simulink model "Model_TranslationEngine64"  (R2022b)
settings: Solver=FixedStepDiscrete  StartTime=0.0  StopTime=5  RelTol=1e-3  EnableMultiTasking=on
InitFcn:
  | % Initialize model
  | ModelSettings=BTConfig.GetModelSettings();
  | 
  | ModelSettings.Validate();
  | 
  | ModelInit;
  | 
  | 
  | % load library data
  | GainLibrary_data;
  | % Load saved values from partition process
  | CapturedConstMask.LoadMapFromFile(bdroot)
StartFcn:
  | % make sure all the simulated RTC requests are found
  | %RTC_SIM_OBJ.ValidateREQs();
undefined symbols (not defined in the file or in its folder): AA, BPLP, Column, NumHFRefBPF, NumHFRefLPF, NumMusicChannels, Row, VolumeMuteConfig
libraries: TuneVar x925, TOP x490, FeaturePath x111, CapturedConstLib x52
(part 33 of 34)

== matlab function Model_TranslationEngine64/ModelPreAmp/DecRate/AudioPilot35/Audiopilot_3_5/GainCalculation/Boosts/DownwardExpansionOn/BassEnable ==
  data: on input; slopeOut output; slope input
  events: trigger input FUNCTION_CALL_EVENT
function slopeOut  = enable(on,slope)
%#codegen
slopeOut = slope.Value * on.Value;

== matlab function Model_TranslationEngine64/ModelPreAmp/DecRate/AudioPilot35/Audiopilot_3_5/GainCalculation/Boosts/DownwardExpansionOn/MidrangeEnable ==
  data: on input; slopeOut output; slope input
  events: trigger input FUNCTION_CALL_EVENT
function slopeOut  = enable(on,slope)
%#codegen
slopeOut = slope.Value * on.Value;

== matlab function Model_TranslationEngine64/ModelPreAmp/DecRate/AudioPilot35/Audiopilot_3_5/GainApplication/Compensation/MidrangeLpfAlignDelay/AlignDelay/MaxCheck ==
  data: DelaySamples input; MaxDelaySamples input; Samples output
  events: trigger input FUNCTION_CALL_EVENT
function Samples = fcn(DelaySamples, MaxDelaySamples)
% Check that number of delay samples will not exceed allotted delay buffer

%Check against the max
if DelaySamples.Value > MaxDelaySamples
    TranslateError('Delay amount cannot be greater than specified max delay');
end

Samples = DelaySamples.Value;

== matlab function Model_TranslationEngine64/ModelPreAmp/DecRate/AudioPilot35/Audiopilot_3_5/GainCalculation/Boosts/DownwardExpansionOn/TrebleEnable ==
  data: on input; slopeOut output; slope input
  events: trigger input FUNCTION_CALL_EVENT
function slopeOut  = enable(on,slope)
%#codegen
slopeOut = slope.Value * on.Value;

== matlab function Model_TranslationEngine64/ModelPreAmp/DecRate/AudioPilot35/Audiopilot_3_5/GainCalculation/Boosts/DyneqOn/DynEqEnable ==
  data: slopeOut output; slope input; on input
  events: trigger input FUNCTION_CALL_EVENT
function slopeOut  = enable(slope,on)
%#codegen
slopeOut = slope.Value * on.Value;

== matlab function Model_TranslationEngine64/ModelPreAmp/DecRate/AudioPilot35/Audiopilot_3_5/NoiseEstimationVariant/RegularNoiseEstimation/LFNoiseEstimatorCoh/LfPreProcess/FilterMic/InnerLink/PoolIirTunableWithReset/Translation ==
  data: RawSOS input; NumStages input; PoolNumStages output; PoolCoeffs output; MaxNumStages parameter; VariantUint8 parameter; NumChannels input
  events: trigger input FUNCTION_CALL_EVENT
function [PoolNumStages, PoolCoeffs] = pooliirTranslation(RawSOS, NumStages, MaxNumStages, VariantUint8,  NumChannels)
%#codegen

% Translation from raw SOS for pool SOS

% Some build time sanity size checking before calling the translation
if numel(NumStages.Value) ~= NumChannels
    error('Size of num stages has to match number of input channels')
end

if RawSOS.Size(2) ~= 6
    error ('Coefficient pool matrix must have 6 columns')
end

[PoolNumStages, PoolCoeffs] = poolIirTranslation(RawSOS, NumStages, MaxNumStages, VariantUint8);

% VariantStr = char(VariantUint8);
% switch (VariantStr)
%     case {"Generic","SharcPlusCore"}
%         % These variants order biquad coefficients in a compacted form
%         [PoolNumStages, PoolCoeffs] = pooliirTranslationFcn(RawSOS, NumStages, MaxNumStages);
%     case {"SharcPlusAccelGul","SharcPlusAccelGxp"}
%         % These variants order biquad coefficients for the ADI accelerator
%         [PoolNumStages, PoolCoeffs] = pooliirAccelTranslationFcn(RawSOS, NumStages, MaxNumStages);
%     case{"Hexagon"}
%         % Hexagon specific order for biquad coefficients 
%         [PoolNumStages, PoolCoeffs] = PoolIirHexagonTranslationFcn(RawSOS, NumStages, MaxNumStages);
%     case{"ArmNeonV7V8"}
%         [PoolNumStages, PoolCoeffs] = PoolIirArmNeonV7V8TranslationFcn(RawSOS, NumStages, MaxNumStages);
%     otherwise
%         % This is a build-time error, not a translation error. The
%         % selected build-time variant is not supported for translation
%         error('Invalid implementation type: [%s]', VariantStr);
% end

end

== matlab function Model_TranslationEngine64/ModelPreAmp/DecRate/AudioPilot35/Audiopilot_3_5/NoiseEstimationVariant/RegularNoiseEstimation/LFNoiseEstimatorCoh/LfPreProcess/FilterRef/InnerLink/PoolIirTunableWithReset/Translation ==
  data: RawSOS input; NumStages input; PoolNumStages output; PoolCoeffs output; MaxNumStages parameter; VariantUint8 parameter; NumChannels input
  events: trigger input FUNCTION_CALL_EVENT
function [PoolNumStages, PoolCoeffs] = pooliirTranslation(RawSOS, NumStages, MaxNumStages, VariantUint8,  NumChannels)
%#codegen

% Translation from raw SOS for pool SOS

% Some build time sanity size checking before calling the translation
if numel(NumStages.Value) ~= NumChannels
    error('Size of num stages has to match number of input channels')
end

if RawSOS.Size(2) ~= 6
    error ('Coefficient pool matrix must have 6 columns')
end

[PoolNumStages, PoolCoeffs] = poolIirTranslation(RawSOS, NumStages, MaxNumStages, VariantUint8);

% VariantStr = char(VariantUint8);
% switch (VariantStr)
%     case {"Generic","SharcPlusCore"}
%         % These variants order biquad coefficients in a compacted form
%         [PoolNumStages, PoolCoeffs] = pooliirTranslationFcn(RawSOS, NumStages, MaxNumStages);
%     case {"SharcPlusAccelGul","SharcPlusAccelGxp"}
%         % These variants order biquad coefficients for the ADI accelerator
%         [PoolNumStages, PoolCoeffs] = pooliirAccelTranslationFcn(RawSOS, NumStages, MaxNumStages);
%     case{"Hexagon"}
%         % Hexagon specific order for biquad coefficients 
%         [PoolNumStages, PoolCoeffs] = PoolIirHexagonTranslationFcn(RawSOS, NumStages, MaxNumStages);
%     case{"ArmNeonV7V8"}
%         [PoolNumStages, PoolCoeffs] = PoolIirArmNeonV7V8TranslationFcn(RawSOS, NumStages, MaxNumStages);
%     otherwise
%         % This is a build-time error, not a translation error. The
%         % selected build-time variant is not supported for translation
%         error('Invalid implementation type: [%s]', VariantStr);
% end

end

== matlab function Model_TranslationEngine64/ModelPreAmp/DecRate/AudioPilot35/Audiopilot_3_5/GainCalculation/RampedEnable/EnableRampCoef/tau2coef ==
  data: Coef output; Tau input; FrameRate parameter
  events: trigger input FUNCTION_CALL_EVENT
function Coef  = fcn(Tau,FrameRate)
% Convert time constant into filter coefficient
%#codegen

Coef = (1 - sin(1/(Tau.Value * FrameRate))) ...
    / cos(1/(Tau.Value * FrameRate));

== matlab function Model_TranslationEngine64/ModelPreAmp/DecRate/AudioPilot35/EntertainmentLevelDetection/AudiopilotLevelDetect/AudiopilotLevelDetect/SlowDecay/sec2samples ==
  data: y output; u input; FrameRate parameter
  events: trigger input FUNCTION_CALL_EVENT
function y  = fcn(u,FrameRate)
%#codegen

y = -abs(u.Value/FrameRate);

== matlab function Model_TranslationEngine64/ModelPreAmp/DecRate/AudioPilot35/Audiopilot_3_5/NoiseEstimationVariant/RegularNoiseEstimation/HFNoiseEstimatorCoh/HfNoiseMusicSeparation /RefPowerMin/undB ==
  data: TOP output; Tune input
  events: trigger input FUNCTION_CALL_EVENT
function TOP  = fcn(Tune)
%#codegen

TOP = undb20(Tune.Value);

== matlab function Model_TranslationEngine64/ModelPreAmp/DecRate/AudioPilot35/Audiopilot_3_5/NoiseEstimationVariant/RegularNoiseEstimation/LFNoiseEstimatorCoh/SpeedBoundsAndNoiseSlew/SpeedBounds/min/Trivial Translation ==
  data: TOP output; Tune1 input; minBoundsLowestVal output
  events: trigger input FUNCTION_CALL_EVENT
function [TOP, minBoundsLowestVal]  = fcn(Tune1)
%#codegen

TOP = Tune1.Value;
minBoundsLowestVal = min(Tune1.Value);

== matlab function Model_TranslationEngine64/ModelPreAmp/DecRate/AudioPilot35/Audiopilot_3_5/NoiseEstimationVariant/RegularNoiseEstimation/HFNoiseEstimatorCoh/PostProcessing/HfImpulseRejection/MinSearch/SubWinLen/Sec2Samples ==
  data: samples output; time input; HFDecRate2 parameter
  events: trigger input FUNCTION_CALL_EVENT
function samples  = Sec2Samples(time,HFDecRate2)
% Convert period in sec to samples
%#codegen

samples = ceil(HFDecRate2*time.Value);

== matlab function Model_TranslationEngine64/ModelPreAmp/DecRate/AudioPilot35/Audiopilot_3_5/NoiseEstimationVariant/RegularNoiseEstimation/HFNoiseEstimatorCoh/PostProcessing/HfSlew/attack/sec2sample ==
  data: u input; y output; HFDecRate2 parameter
  events: trigger input FUNCTION_CALL_EVENT
function y = fcn(u, HFDecRate2)
% Convert rate from per sec to per sample

y = (u.Value/HFDecRate2);

== matlab function Model_TranslationEngine64/ModelPreAmp/DecRate/AudioPilot35/Audiopilot_3_5/NoiseEstimationVariant/RegularNoiseEstimation/HFNoiseEstimatorCoh/PostProcessing/HfSlew/decay/sec2sample ==
  data: u input; y output; HFDecRate2 parameter
  events: trigger input FUNCTION_CALL_EVENT
function y = fcn(u, HFDecRate2)
% Convert rate from per sec to per sample

y = -abs(u.Value/HFDecRate2);

== matlab function Model_TranslationEngine64/ModelPreAmp/DecRate/AudioPilot35/Audiopilot_3_5/NoiseEstimationVariant/RegularNoiseEstimation/HFNoiseEstimatorCoh/ReferenceLatency/RefLatency/ms2samples ==
  data: DelayTimeMS input; MaxLatencySamples input; Samples output; HFDecRate parameter
  events: trigger input FUNCTION_CALL_EVENT
function Samples = fcn(DelayTimeMS, MaxLatencySamples, HFDecRate)
% Convert from time constant to samples

Samples = floor(DelayTimeMS.Value*HFDecRate/1000);
% Use floor to minimize the risk of going noncausal 

if Samples > MaxLatencySamples
    TranslateError('Delay amount cannot be greater than specified max delay');
end

== matlab function Model_TranslationEngine64/ModelPreAmp/DecRate/AudioPilot35/Audiopilot_3_5/NoiseEstimationVariant/RegularNoiseEstimation/LFNoiseEstimatorCoh/LfNoiseImpulseRejection/Gamma0/TimeConstant2Coefficient ==
  data: coef output; tau input; DecRate3 parameter
  events: trigger input FUNCTION_CALL_EVENT
function coef  = fcn(tau,DecRate3)
% Convert time constant to filter coefficient
%#codegen

wc = 1/(DecRate3*tau.Value);
coef = (1-sin(wc))/cos(wc);

== matlab function Model_TranslationEngine64/ModelPreAmp/DecRate/AudioPilot35/Audiopilot_3_5/NoiseEstimationVariant/RegularNoiseEstimation/RatioCalculation/APLFUP/FlagHoldTime/sec2samples ==
  data: samples output; time input; HFDecRate parameter
  events: trigger input FUNCTION_CALL_EVENT
function samples  = fcn(time,HFDecRate)
%#codegen

samples = ceil(time.Value*HFDecRate);

== matlab function Model_TranslationEngine64/ModelPreAmp/DecRate/AudioPilot35/Audiopilot_3_5/NoiseEstimationVariant/RegularNoiseEstimation/RatioCalculation/APLFUP/LfNoiseUpdatePeriod/sec2samples ==
  data: samples output; time input; HFDecRate parameter
  events: trigger input FUNCTION_CALL_EVENT
function samples = fcn(time,HFDecRate)

% A trivial pass-through translation looks like this:
samples = ceil(time.Value*HFDecRate);

== matlab function Model_TranslationEngine64/ModelPreAmp/DecRate/AudioPilot35/Audiopilot_3_5/NoiseEstimationVariant/RegularNoiseEstimation/LFNoiseEstimatorCoh/LfNoiseImpulseRejection/ImpulseVarianceFilterCoef/TimeConstant2Coefficient ==
  data: coef output; tau input; DecRate3 parameter
  events: trigger input FUNCTION_CALL_EVENT
function coef  = fcn(tau,DecRate3)
% Convert time constant to filter coefficient
%#codegen

wc = 1/(DecRate3*tau.Value);
coef = (1-sin(wc))/cos(wc);

== matlab function Model_TranslationEngine64/ModelPreAmp/DecRate/AudioPilot35/Audiopilot_3_5/NoiseEstimationVariant/RegularNoiseEstimation/RatioCalculation/EnergyLpfCoef/Tau2Coef ==
  data: coef output; tau input; HFDecRate parameter
  events: trigger input FUNCTION_CALL_EVENT
function coef  = Tau2Coef(tau,HFDecRate)
% Convert from time constant to 1st order coefficient
%#codegen

wc = 1/(HFDecRate*tau.Value);
coef = (1-sin(wc))/cos(wc);

== matlab function Model_TranslationEngine64/ModelPreAmp/DecRate/AudioPilot35/Audiopilot_3_5/NoiseEstimationVariant/RegularNoiseEstimation/RatioCalculation/RatioSlew/attack/sec2sample ==
  data: u input; y output; HFDecRate parameter
  events: trigger input FUNCTION_CALL_EVENT
function y = fcn(u, HFDecRate)
% Convert rate from per sec to per sample

y = abs(u.Value/HFDecRate);

== matlab function Model_TranslationEngine64/ModelPreAmp/DecRate/AudioPilot35/Audiopilot_3_5/NoiseEstimationVariant/RegularNoiseEstimation/RatioCalculation/RatioSlew/decay/sec2sample ==
  data: u input; y output; HFDecRate parameter
  events: trigger input FUNCTION_CALL_EVENT
function y = RateConversion(u, HFDecRate)
% Convert rate from per sec to per sample

y = -abs(u.Value/HFDecRate);

== matlab function Model_TranslationEngine64/ModelPreAmp/DecRate/AudioPilot35/Audiopilot_3_5/NoiseEstimationVariant/RegularNoiseEstimation/RatioCalculation/RatioSmoother/RatioImpulseRejectionGamma0/Tau2Gamma ==
  data: gamma output; tau input; HFDecRate parameter
  events: trigger input FUNCTION_CALL_EVENT
function gamma  = Tau2Gamma(tau,HFDecRate)
% Approximate conversion from coefficient to time constant

wc = 1/(HFDecRate*tau.Value);
gamma = 1-(1-sin(wc))/cos(wc);

== matlab function Model_TranslationEngine64/ModelPreAmp/DecRate/AudioPilot35/Audiopilot_3_5/NoiseEstimationVariant/RegularNoiseEstimation/LFNoiseEstimatorCoh/ReferenceLatency/RefLatencySamples/ms2samples ==
  data: DelayTimeMS input; MaxLatencySamples input; Samples output; DecRate parameter
  events: trigger input FUNCTION_CALL_EVENT
function Samples = fcn(DelayTimeMS, MaxLatencySamples, DecRate)
% Convert from milliseconds to samples

% Use floor to minimize the risk of going noncausal 
Samples = floor(DelayTimeMS.Value*DecRate/1000);


if Samples > MaxLatencySamples
    TranslateError('Delay amount cannot be greater than specified max delay');
end

== matlab function Model_TranslationEngine64/ModelPreAmp/DecRate/AudioPilot35/Audiopilot_3_5/NoiseEstimationVariant/RegularNoiseEstimation/LFNoiseEstimatorCoh/SpeedBoundsAndNoiseSlew/LfNoiseSlew/Attack/sec2sample ==
  data: u input; y output; DecRate2 parameter
  events: trigger input FUNCTION_CALL_EVENT
function y = fcn(u, DecRate2)
% Convert rate from per second to per sample

y = u.Value/DecRate2;

== matlab function Model_TranslationEngine64/ModelPreAmp/DecRate/AudioPilot35/Audiopilot_3_5/NoiseEstimationVariant/RegularNoiseEstimation/LFNoiseEstimatorCoh/SpeedBoundsAndNoiseSlew/LfNoiseSlew/Decay/sec2sample ==
  data: u input; y output; DecRate2 parameter
  events: trigger input FUNCTION_CALL_EVENT
function y = fcn(u, DecRate2)
% Convert rate from per second to per sample

y = -abs(u.Value/DecRate2);

== matlab function Model_TranslationEngine64/ModelPreAmp/DecRate/AudioPilot35/Audiopilot_3_5/NoiseEstimationVariant/RegularNoiseEstimation/LFNoiseEstimatorCoh/SpeedBoundsAndNoiseSlew/LfNoiseSlew/SlowSlew/sec2sample ==
  data: u input; y output; DecRate2 parameter
  events: trigger input FUNCTION_CALL_EVENT
function y = fcn(u, DecRate2)
% Convert rate from per second to per sample

y = u.Value/DecRate2;

== matlab function Model_TranslationEngine64/ModelPreAmp/DecRate/AudioPilot35/Audiopilot_3_5/NoiseEstimationVariant/RegularNoiseEstimation/RatioCalculation/RatioSmoother/RatioImpulseRejectionImpulseVarianceLpfCoef/Tau2Coef ==
  data: coef output; tau input; HFDecRate parameter
  events: trigger input FUNCTION_CALL_EVENT
function coef  = Tau2Coef(tau,HFDecRate)
% Convert from time constant to 1st order coefficient
%#codegen

wc = 1/(HFDecRate*tau.Value);
coef = (1-sin(wc))/cos(wc);

== matlab function Model_TranslationEngine64/ModelPreAmp/DecRate/AudioPilot35/EntertainmentLevelDetection/PreProcessing/PreEmphasisShelfFilter/InnerLink/PoolIirTunableWithReset/Translation ==
  data: RawSOS input; NumStages input; PoolNumStages output; PoolCoeffs output; MaxNumStages parameter; VariantUint8 parameter; NumChannels input
  events: trigger input FUNCTION_CALL_EVENT
function [PoolNumStages, PoolCoeffs] = pooliirTranslation(RawSOS, NumStages, MaxNumStages, VariantUint8,  NumChannels)
%#codegen

% Translation from raw SOS for pool SOS

% Some build time sanity size checking before calling the translation
if numel(NumStages.Value) ~= NumChannels
    error('Size of num stages has to match number of input channels')
end

if RawSOS.Size(2) ~= 6
    error ('Coefficient pool matrix must have 6 columns')
end

[PoolNumStages, PoolCoeffs] = poolIirTranslation(RawSOS, NumStages, MaxNumStages, VariantUint8);

% VariantStr = char(VariantUint8);
% switch (VariantStr)
%     case {"Generic","SharcPlusCore"}
%         % These variants order biquad coefficients in a compacted form
%         [PoolNumStages, PoolCoeffs] = pooliirTranslationFcn(RawSOS, NumStages, MaxNumStages);
%     case {"SharcPlusAccelGul","SharcPlusAccelGxp"}
%         % These variants order biquad coefficients for the ADI accelerator
%         [PoolNumStages, PoolCoeffs] = pooliirAccelTranslationFcn(RawSOS, NumStages, MaxNumStages);
%     case{"Hexagon"}
%         % Hexagon specific order for biquad coefficients 
%         [PoolNumStages, PoolCoeffs] = PoolIirHexagonTranslationFcn(RawSOS, NumStages, MaxNumStages);
%     case{"ArmNeonV7V8"}
%         [PoolNumStages, PoolCoeffs] = PoolIirArmNeonV7V8TranslationFcn(RawSOS, NumStages, MaxNumStages);
%     otherwise
%         % This is a build-time error, not a translation error. The
%         % selected build-time variant is not supported for translation
%         error('Invalid implementation type: [%s]', VariantStr);
% end

end

== matlab function Model_TranslationEngine64/ModelPreAmp/DecRate/Medusa5H1/Balance/Balance/TuneVarTable/Balance_Table_Translation ==
  data: tableDb output; tableIdx output; balanceTable input
  events: trigger input FUNCTION_CALL_EVENT
function [tableDb, tableIdx] = fcn(balanceTable)
%#codegen

% Set up the size and datatype of our TOP outputs:
maxTableSize = numel(balanceTable.Value) / 2;
idxType = 'uint8';
idxStorageType = 'uint32';
dbType = 'single';
tableIdx = zeros(1,maxTableSize,idxStorageType);
tableDb = zeros(1,maxTableSize,dbType);

% separate the pairs into their index and value components
givenPairs = balanceTable.Size(1);
indexes = balanceTable.Value(1:givenPairs,1);
values = balanceTable.Value(1:givenPairs,2);

% then sort and ignore duplicates
[cleanIdx,map] = unique(indexes);

% Validate input sizes
numPairs = numel(map);
argName='BalanceTable';

% Validate: enough data?
if (numPairs < 2)
    TranslateError('%s must have at least 2 index pairs. Encounted value with only %f pairs\n', argName, numPairs);
end

% Validate: Highest index still below 255?
if (cleanIdx(1) < 0 || cleanIdx(end) > intmax(idxType))
    TranslateError('%s out of range table index %f encountered. Index must be between 0 and %d.\n',argName,cleanIdx(end),intmax(idxType));
end

% fill in the table buffer with provided pairs
tableIdx(1:numPairs) = cleanIdx(1:numPairs);
tableDb(1:numPairs) = values(map(1:numPairs));

% fill the rest of the table buffer with the last entry
remainingPairs = numel(map)+1:maxTableSize;
tableIdx(remainingPairs) = tableIdx(numPairs);
tableDb(remainingPairs) =  tableDb(numPairs);

end

== matlab function Model_TranslationEngine64/ModelPreAmp/DecRate/Medusa5H1/MedusaHoligram/Medusa5H1 Part 1/Bass Manager Stereo/Bass Manager Tuning/translation ==
  data: LeftMixWeights output; SurroundOn input; LeftMixWeightsIn input; RightMixWeightsIn input; RightMixWeights output; NumInputs parameter
  events: trigger input FUNCTION_CALL_EVENT
function [LeftMixWeights, RightMixWeights]  = fcn(SurroundOn, LeftMixWeightsIn, RightMixWeightsIn, NumInputs)
% Expected Order of Weights:
% LeftMixWeightsIn = [L2L, Ls2L, Ltf2L, Ltb2L, C2L, Lfe2L]
% RightMixWeightsIn = [R2R, Rs2R, Rtf2R, Rtb2R, C2R, Lfe2R]

if (SurroundOn.Value == 3 || SurroundOn.Value == 4)
    % Mix weights are only applicable for 5.1 and 5.1.4 inputs

    % Check if any of the tuned mix weights are negative
    if(sum(LeftMixWeightsIn.Value < 0))
        TranslateError('Medusa Bass Manager: Left mix weights cannot be less than 0.');
    end

    if(sum(RightMixWeightsIn.Value < 0))
        TranslateError('Medusa Bass Manager: Right mix weights cannot be less than 0.');
    end

    % Cast the mix weights to 'single' data type
    LeftMixWeights = single(LeftMixWeightsIn.Value);
    RightMixWeights = single(RightMixWeightsIn.Value);

    if(SurroundOn.Value == 3 && NumInputs == 10)
        % For 5.1 input, set weights corresponding to heigh channels to 0
        % Ltf2L = 0
        % Ltb2L = 0
        % Rtf2R = 0
        % Rtb2R = 0
        LeftMixWeights(3:4) = [0 0];
        RightMixWeights(3:4) = [0 0];
    end

else
    % For 2-channel input, use pre-defined weights to enable pass-through
    % L2L = 1.0
    % R2R = 1.0
    % All other combinations are set to 0

    % Extracting the dimension of MixWeights
    NumMixWeights = size(LeftMixWeightsIn.Value);
    
    LeftMixWeights = single(eye(NumMixWeights));
    RightMixWeights = single(eye(NumMixWeights)); 

end

== matlab function Model_TranslationEngine64/ModelPreAmp/DecRate/Medusa5H1/MedusaHoligram/Medusa5H1 Part 2/Alignment Delay/Full-rate Alignment Delay Translation/translation ==
  data: wiggleDelay input; NEARWiggleDelay input; holigramDelay input; trebleDelay output; DecimationFactor parameter; DeciRateMaxWiggleDelay parameter; DeciRateMaxNearWiggleDelay parameter; MaxHoligramDelay parameter; DeciRateFdpDelay parameter; FullRateFdpDelay parameter; MaxTrebleDelay parameter
  events: trigger input FUNCTION_CALL_EVENT
function trebleDelay   = fcn(wiggleDelay, NEARWiggleDelay, holigramDelay,...
                                DecimationFactor, DeciRateMaxWiggleDelay,...
                                DeciRateMaxNearWiggleDelay, MaxHoligramDelay,...
                                DeciRateFdpDelay, FullRateFdpDelay, MaxTrebleDelay)
%#codegen
%[Param:DecimationFactor]
%[Param:DeciRateMaxWiggleDelay]
%[Param:DeciRateMaxNearWiggleDelay]
%[Param:MaxHoligramDelay]
%[Param:DeciRateFdpDelay]
%[Param:FullRateFdpDelay]
%[Param:MaxTrebleDelay]

%% Treble Delay Translation
% This translation computes the alignment delay values for full-rate
% upmixed components

% Extracting build-time parameters from config struct
DEC = DecimationFactor;

%% Error Check for incoming tune values
if(wiggleDelay.Value < 0)
    TranslateError('Value of ''Medusa Wiggle Delay'' must be greater than or equal to zero.');
end

if(NEARWiggleDelay.Value < 0)
    TranslateError('Value of ''NEAR Wiggle Delay'' must be greater than or equal to zero.');
end

if(holigramDelay.Value < 0)
    TranslateError('Value of ''Medusa Holigram Delay'' must be greater than or equal to zero.');
end

if(wiggleDelay.Value > DeciRateMaxWiggleDelay)
    TranslateError('Value of ''Medusa Wiggle Delay'' must be less than or equal to %d.', DeciRateMaxWiggleDelay);
end

if(NEARWiggleDelay.Value > DeciRateMaxNearWiggleDelay)
    TranslateError('Value of ''NEAR Wiggle Delay'' must be less than or equal to %d.', DeciRateMaxNearWiggleDelay);
end

if(holigramDelay.Value > MaxHoligramDelay)
    TranslateError('Value of ''Medusa Holigram Delay'' must be less than or equal to %d.', MaxHoligramDelay);
end

%% Computing the alignment delay values for treble path
% Medusa wiggle filter latency
wiggleDelayDec = int32(round(wiggleDelay.Value));
wiggleDelayFull = int32(wiggleDelayDec * DEC);

% NEAR wiggle filter latency
NEARWiggleDelayDec = int32(round(NEARWiggleDelay.Value));
NEARWiggleDelayFull = int32(NEARWiggleDelayDec * DEC);

% Holigram filter latency
holigramDelayFull = int32(round(holigramDelay.Value));

% Compute the treble alignment delay (applies to full-rate upmixed components)
actualTrebleDelay = DeciRateFdpDelay - FullRateFdpDelay + wiggleDelayFull + NEARWiggleDelayFull + holigramDelayFull;

%% Error check for outgoing alignment delay value
if(actualTrebleDelay > MaxTrebleDelay)
   TranslateError('Value of ''Medusa Treble Delay'' on full-rate path exceeds the maximum value of %d.', MaxTrebleDelay);
end

%% Assigning output
trebleDelay = actualTrebleDelay;

end

== matlab function Model_TranslationEngine64/ModelPreAmp/DecRate/AudioPilot35/EntertainmentLevelDetection/DyneqLevelDetect/DyneqLevelDetect/FastDecay/sec2samples ==
  data: y output; u input; FrameRate parameter
  events: trigger input FUNCTION_CALL_EVENT
function y  = fcn(u,FrameRate)
%#codegen

y = -abs(u.Value/FrameRate);

== matlab function Model_TranslationEngine64/ModelPreAmp/DecRate/AudioPilot35/EntertainmentLevelDetection/DyneqLevelDetect/DyneqLevelDetect/HoldMargin/SetPositive ==
  data: TOP output single; Tune input
  events: trigger input FUNCTION_CALL_EVENT
function TOP = fcn(Tune)
%#codegen

TOP = abs(Tune.Value);

== matlab function Model_TranslationEngine64/ModelPreAmp/DecRate/AudioPilot35/EntertainmentLevelDetection/DyneqLevelDetect/DyneqLevelDetect/HoldTime/sec2samples ==
  data: y output; u input; FrameRate parameter
  events: trigger input FUNCTION_CALL_EVENT
function y  = fcn(u,FrameRate)
%#codegen

y = ceil(u.Value*FrameRate);

== matlab function Model_TranslationEngine64/ModelPreAmp/DecRate/AudioPilot35/EntertainmentLevelDetection/DyneqLevelDetect/DyneqLevelDetect/SlowDecay/sec2samples ==
  data: y output; u input; FrameRate parameter
  events: trigger input FUNCTION_CALL_EVENT
function y  = fcn(u,FrameRate)
%#codegen

y = -abs(u.Value/FrameRate);

== matlab function Model_TranslationEngine64/ModelPreAmp/DecRate/AudioPilot35/Volume/Index2DbTable/table translation ==
  data: Table_Idx output; Table_dB output; Table input
  events: trigger input FUNCTION_CALL_EVENT
function [Table_Idx,Table_dB] = fcn(Table)
%#codegen
%
% Demux table matrix into one dimesional value and index vectors
%
%
% Set up the size and datatype of our TOP outputs:
maxTableSize = numel(Table.Value) / 2;
idxType = 'uint8';
idxStorageType = 'uint32';
dbType = 'single';
Table_Idx = zeros(1,maxTableSize,idxStorageType);
Table_dB = zeros(1,maxTableSize,dbType);

% separate the pairs into their index and value components
givenPairs = Table.Size(1);
indexes = Table.Value(1:givenPairs,1);
values = Table.Value(1:givenPairs,2);

% then sort and ignore duplicates
[cleanIdx,map] = unique(indexes);

% Validate input sizes
numPairs = numel(map);
argName='Table';

% Validate: enough data?
if (numPairs < 2)
    TranslateError('%s must have at least 2 index pairs. Encounted value with only %f pairs\n', argName, numPairs);
end

% Validate: Highest index still below 1.0?
if (cleanIdx(end) > 1)
    TranslateError('%s out of range table index %f encountered. Index must be between 0 and 1.\n',argName,cleanIdx(end));
end

% fill in the table buffer with provided pairs
for i=1:numPairs
    Table_Idx(i) = intmax(idxType) * cleanIdx(i);
    Table_dB(i) = values(map(i));
end
% fill the rest of the table buffer with the last entry
for j=numel(map)+1:maxTableSize
    Table_Idx(j) = Table_Idx(numPairs);
    Table_dB(j) =  Table_dB(numPairs);
end

end

== matlab function Model_TranslationEngine64/ModelPreAmp/DecRate/Medusa5H1/MedusaHoligram/Medusa5H1 Part 2/SPUM Decay Estimate/High-pass filter > 6kHz/InnerLink/PoolIirTunableWithReset/Translation ==
  data: RawSOS input; NumStages input; PoolNumStages output; PoolCoeffs output; MaxNumStages parameter; VariantUint8 parameter; NumChannels input
  events: trigger input FUNCTION_CALL_EVENT
function [PoolNumStages, PoolCoeffs] = pooliirTranslation(RawSOS, NumStages, MaxNumStages, VariantUint8,  NumChannels)
%#codegen

% Translation from raw SOS for pool SOS

% Some build time sanity size checking before calling the translation
if numel(NumStages.Value) ~= NumChannels
    error('Size of num stages has to match number of input channels')
end

if RawSOS.Size(2) ~= 6
    error ('Coefficient pool matrix must have 6 columns')
end

[PoolNumStages, PoolCoeffs] = poolIirTranslation(RawSOS, NumStages, MaxNumStages, VariantUint8);

% VariantStr = char(VariantUint8);
% switch (VariantStr)
%     case {"Generic","SharcPlusCore"}
%         % These variants order biquad coefficients in a compacted form
%         [PoolNumStages, PoolCoeffs] = pooliirTranslationFcn(RawSOS, NumStages, MaxNumStages);
%     case {"SharcPlusAccelGul","SharcPlusAccelGxp"}
%         % These variants order biquad coefficients for the ADI accelerator
%         [PoolNumStages, PoolCoeffs] = pooliirAccelTranslationFcn(RawSOS, NumStages, MaxNumStages);
%     case{"Hexagon"}
%         % Hexagon specific order for biquad coefficients 
%         [PoolNumStages, PoolCoeffs] = PoolIirHexagonTranslationFcn(RawSOS, NumStages, MaxNumStages);
%     case{"ArmNeonV7V8"}
%         [PoolNumStages, PoolCoeffs] = PoolIirArmNeonV7V8TranslationFcn(RawSOS, NumStages, MaxNumStages);
%     otherwise
%         % This is a build-time error, not a translation error. The
%         % selected build-time variant is not supported for translation
%         error('Invalid implementation type: [%s]', VariantStr);
% end

end

== matlab function Model_TranslationEngine64/ModelPreAmp/DecRate/Medusa5H1/Balance/Balance/channel_ramper_translation ==
  data: ChanRampMap output; TuneChanRampMap input; channelCount input; MaskNumRampers parameter
  events: trigger input FUNCTION_CALL_EVENT
function ChanRampMap  = fcn(TuneChanRampMap, channelCount, ... % inputs
    MaskNumRampers) % parameters

% Verifies if each channel is assigned to one of the 4 possible rampers. 
% Acceptable rampers:
% 1: left
% 2: right
% 3: center
% 4: unused

argName = 'Balance';

% Ensure each channel is present in the map
inputMapWidth = numel(TuneChanRampMap.Value);
if (inputMapWidth ~= channelCount)
   error(['Error in %s : Channel-to-ramper map width [%d] does not match number of ',...
       'audio channels [%d]. Make sure all channels are assigned ',...
       'to either the left or right groups.'], argName, inputMapWidth, ...
       channelCount);
end

% Verify that the channels are assigned to valid group numbers.

if (numel(unique(TuneChanRampMap.Value)) > (MaskNumRampers + 1))
    error(['Error in [%s] : Atleast 1 channel has been assigned to the incorrect group.' ...
        'Group numbers assigned to channels in the Channel-to-ramper '...
        'map should be a number between 1 and 4, corresponding to one '...
        'of the 4 possible speaker contents .'], argName);        
end

if (sum(TuneChanRampMap.Value == 0) > 0)
   error(['Error in [%s] : Valid ramper values for the channel to '...
       'ramper map must be between 1 and 4, or "-1" to indicate an '... 
       'unused channel .'], argName);
end

ChanRampMap = int32(TuneChanRampMap.Value);

== matlab function Model_TranslationEngine64/ModelPreAmp/DecRate/Medusa5H1/MedusaHoligram/Medusa5H1 Part 1/Bass Manager Stereo/HPF/PoolIirTunableWithReset/Translation ==
  data: RawSOS input; NumStages input; PoolNumStages output; PoolCoeffs output; MaxNumStages parameter; VariantUint8 parameter; NumChannels input
  events: trigger input FUNCTION_CALL_EVENT
function [PoolNumStages, PoolCoeffs] = pooliirTranslation(RawSOS, NumStages, MaxNumStages, VariantUint8,  NumChannels)
%#codegen

% Translation from raw SOS for pool SOS

% Some build time sanity size checking before calling the translation
if numel(NumStages.Value) ~= NumChannels
    error('Size of num stages has to match number of input channels')
end

if RawSOS.Size(2) ~= 6
    error ('Coefficient pool matrix must have 6 columns')
end

[PoolNumStages, PoolCoeffs] = poolIirTranslation(RawSOS, NumStages, MaxNumStages, VariantUint8);

% VariantStr = char(VariantUint8);
% switch (VariantStr)
%     case {"Generic","SharcPlusCore"}
%         % These variants order biquad coefficients in a compacted form
%         [PoolNumStages, PoolCoeffs] = pooliirTranslationFcn(RawSOS, NumStages, MaxNumStages);
%     case {"SharcPlusAccelGul","SharcPlusAccelGxp"}
%         % These variants order biquad coefficients for the ADI accelerator
%         [PoolNumStages, PoolCoeffs] = pooliirAccelTranslationFcn(RawSOS, NumStages, MaxNumStages);
%     case{"Hexagon"}
%         % Hexagon specific order for biquad coefficients 
%         [PoolNumStages, PoolCoeffs] = PoolIirHexagonTranslationFcn(RawSOS, NumStages, MaxNumStages);
%     case{"ArmNeonV7V8"}
%         [PoolNumStages, PoolCoeffs] = PoolIirArmNeonV7V8TranslationFcn(RawSOS, NumStages, MaxNumStages);
%     otherwise
%         % This is a build-time error, not a translation error. The
%         % selected build-time variant is not supported for translation
%         error('Invalid implementation type: [%s]', VariantStr);
% end

end

== matlab function Model_TranslationEngine64/ModelPreAmp/DecRate/Medusa5H1/MedusaHoligram/Medusa5H1 Part 1/Bass Manager Stereo/LPF/PoolIirTunableWithReset/Translation ==
  data: RawSOS input; NumStages input; PoolNumStages output; PoolCoeffs output; MaxNumStages parameter; VariantUint8 parameter; NumChannels input
  events: trigger input FUNCTION_CALL_EVENT
function [PoolNumStages, PoolCoeffs] = pooliirTranslation(RawSOS, NumStages, MaxNumStages, VariantUint8,  NumChannels)
%#codegen

% Translation from raw SOS for pool SOS

% Some build time sanity size checking before calling the translation
if numel(NumStages.Value) ~= NumChannels
    error('Size of num stages has to match number of input channels')
end

if RawSOS.Size(2) ~= 6
    error ('Coefficient pool matrix must have 6 columns')
end

[PoolNumStages, PoolCoeffs] = poolIirTranslation(RawSOS, NumStages, MaxNumStages, VariantUint8);

% VariantStr = char(VariantUint8);
% switch (VariantStr)
%     case {"Generic","SharcPlusCore"}
%         % These variants order biquad coefficients in a compacted form
%         [PoolNumStages, PoolCoeffs] = pooliirTranslationFcn(RawSOS, NumStages, MaxNumStages);
%     case {"SharcPlusAccelGul","SharcPlusAccelGxp"}
%         % These variants order biquad coefficients for the ADI accelerator
%         [PoolNumStages, PoolCoeffs] = pooliirAccelTranslationFcn(RawSOS, NumStages, MaxNumStages);
%     case{"Hexagon"}
%         % Hexagon specific order for biquad coefficients 
%         [PoolNumStages, PoolCoeffs] = PoolIirHexagonTranslationFcn(RawSOS, NumStages, MaxNumStages);
%     case{"ArmNeonV7V8"}
%         [PoolNumStages, PoolCoeffs] = PoolIirArmNeonV7V8TranslationFcn(RawSOS, NumStages, MaxNumStages);
%     otherwise
%         % This is a build-time error, not a translation error. The
%         % selected build-time variant is not supported for translation
%         error('Invalid implementation type: [%s]', VariantStr);
% end

end

== matlab function Model_TranslationEngine64/ModelPreAmp/DecRate/AudioPilot35/EntertainmentLevelDetection/PreProcessing/MusicDelay/Ms2Samples ==
  data: DelayTimeMs input; MaxLatencySamples input; Samples output; SampleRate parameter
  events: trigger input FUNCTION_CALL_EVENT
function Samples = Ms2Samples(DelayTimeMs, MaxLatencySamples, SampleRate)
% Convert delay time to delay samples
% Check that delay time in msec will not exceed allotted delay buffer

Samples = floor(DelayTimeMs.Value*SampleRate/1000);
% Use floor to minimize the risk of going noncausal 

if Samples > MaxLatencySamples
    TranslateError('Delay amount cannot be greater than specified max delay');
end

== matlab function Model_TranslationEngine64/ModelPreAmp/DecRate/Medusa5H1/MedusaHoligram/Medusa5H1 Part 2/Mono Detector/Mono Detector/Tune Translations/translation ==
  data: LevelPole output; LevelCutoff input; LevelGain output; LSSmoothCutoff input; LSSmoothResetCutoff input; LSSmoothPole output; LSSmoothGain output; LSSmoothResetPole output; LSSmoothResetGain output; FrameRate input
  events: trigger input FUNCTION_CALL_EVENT
function [LevelPole, LevelGain, LSSmoothPole, LSSmoothGain, ...
    LSSmoothResetPole, LSSmoothResetGain] = fcn(LevelCutoff, ...
    LSSmoothCutoff, LSSmoothResetCutoff, FrameRate)

% Cutoff is the inverse of time constant in Hz. So this function
% basically converts reciprocal of time constant to first order iir
% filter coefficient.
% Reference: https://bosecorp.sharepoint.com/sites/ASD3/DSPTeam/Shared%20Documents/DSP_Topics/Comparison%20of%20time%20constant%20conversion%20methods.docx

error = false;
if LevelCutoff.Value <= LSSmoothCutoff.Value
    TranslateError('Least square smoother should smooth more than level smoother');
    error = true;
elseif LSSmoothResetCutoff.Value <= LSSmoothCutoff.Value
    TranslateError('Least square smoother for reset should smooth less than that for normal mode');
    error = true;
end

if (~error)
    wn = 2 * pi * LevelCutoff.Value / FrameRate;
    LevelPole = (1 - sin(wn)) ./ cos(wn);
    LevelGain = 1 - LevelPole;

    wn = 2 * pi * LSSmoothCutoff.Value / FrameRate;
    LSSmoothPole = (1 - sin(wn)) ./ cos(wn);
    LSSmoothGain = 1 - LSSmoothPole;

    wn = 2 * pi * LSSmoothResetCutoff.Value / FrameRate;
    LSSmoothResetPole = (1 - sin(wn)) ./ cos(wn);
    LSSmoothResetGain = 1 - LSSmoothResetPole;
else
    LevelPole = 0;
    LevelGain = 0;
    LSSmoothPole = 0;
    LSSmoothGain = 0;   
    LSSmoothResetPole = 0;
    LSSmoothResetGain = 0;     
end

end

== matlab function Model_TranslationEngine64/ModelPreAmp/DecRate/AudioPilot35/Audiopilot_3_5/GainApplication/Compensation/AntizipperRampLpf/Frequency2Coefficients ==
  data: num output single; Freq input; denom output single; SampleRate parameter
  events: trigger input FUNCTION_CALL_EVENT
function [num,denom] = fcn(Freq,SampleRate)
% Forms the numerator and denominator coefficients
% for a first order filter with the specified
% corner frequency

%#codegen

wc = 2 * pi * Freq.Value / SampleRate;
Coef = (1 - sin(wc)) / cos(wc);

num = 1-Coef ;
denom = [1 -Coef];

== matlab function Model_TranslationEngine64/ModelPreAmp/DecRate/Medusa5H1/MedusaHoligram/Medusa5H1 Part 2/Mono Detector/Mono Detector/Tune Translations/translation1 ==
  data: ThresholdZeroLevel output; NoiseFloordB input
  events: trigger input FUNCTION_CALL_EVENT
function ThresholdZeroLevel  = fcn(NoiseFloordB)
% thresh = 2 * undb20(noiseFloordB)
ThresholdZeroLevel = 2 * (10 ^ (NoiseFloordB.Value / 20));

== matlab function Model_TranslationEngine64/ModelPreAmp/DecRate/Medusa5H1/MedusaHoligram/Medusa5H1 Part 2/Mono Detector/Mono Detector/Tune Translations/translation2 ==
  data: LRMatchTolerance output; LRMatchTolerancedB input
  events: trigger input FUNCTION_CALL_EVENT
function LRMatchTolerance  = fcn(LRMatchTolerancedB)

if (LRMatchTolerancedB.Value < 0 || LRMatchTolerancedB.Value > 0.5)
    TranslateError('Invalid tolerance for left right match');
    LRMatchTolerance = 0;
else
    LRMatchTolerance = 10 ^ (LRMatchTolerancedB.Value / 20);
end

== matlab function Model_TranslationEngine64/ModelPreAmp/DecRate/Medusa5H1/MedusaHoligram/Medusa5H1 Part 2/Mono Detector/Mono Detector/Tune Translations/translation3 ==
  data: ThresholdMono output; ThresholdMonoInput input; ThresholdStereoInput input; ThresholdStereo output
  events: trigger input FUNCTION_CALL_EVENT
function [ThresholdMono, ThresholdStereo] = fcn(ThresholdMonoInput, ThresholdStereoInput)
% The exponent 1/64 is carried over from AR and old bdsp implementation.
% This is designed by Chris Cheng to make the gap between two thresholds
% as small as possible, because in theory they should be almost identical.
% Removing this would still work in theory with a slight change in the 
% output. However as we verify the block against PREQ Simulink model, this
% translation is retained to get a complete match in performance.

if ThresholdMonoInput.Value <= ThresholdStereoInput.Value
    TranslateError('Threshold for mono should be higher than that for stereo');
    ThresholdMono = 0;
    ThresholdStereo = 0;
elseif (ThresholdMonoInput.Value >= 1) || (ThresholdStereoInput.Value >= 1)
    TranslateError('Threshold values for mono and stereo should be less than 1.0');
    ThresholdMono = 0;
    ThresholdStereo = 0;
else
    ThresholdMono = ThresholdMonoInput.Value ^ (1/64);
    ThresholdStereo = ThresholdStereoInput.Value ^ (1/64);
end

== matlab function Model_TranslationEngine64/ModelPreAmp/DecRate/Medusa5H1/MedusaHoligram/Medusa5H1 Part 2/Decimated-Rate FDP/Fdp/FreqDomainProcessing/CalculateAndApplyCoefficients/DeciRate/Calculate coefficients/StretchParamsTuning/Trivial Translation ==
  data: XpMax output; XpMaxIn input; LokRokMaxScaleFactor output; XpMinIn input; XpMin output
  events: trigger input FUNCTION_CALL_EVENT
function [XpMax, LokRokMaxScaleFactor,  XpMin] = fcn(XpMaxIn, XpMinIn)

XpMax = XpMaxIn.Value;
XpMin = XpMinIn.Value;
if (XpMin < 0) || (XpMin >= 1)
    TranslateError('XpMin must be no less than 0.0, and must be less than 1.0');
end

if (XpMax < 0) || (XpMax >= 1)
    TranslateError('XpMax must be no less than 0.0, and must be less than 1.0');
end

if (XpMax < XpMin)
    TranslateError('XpMin cannot exceed XpMax');
end

if (XpMax == 1)
    LokRokMaxScaleFactor = 0;
else
    LokRokMaxScaleFactor = 0.5 * XpMax / (1 - XpMax);
end

end

== matlab function Model_TranslationEngine64/ModelPreAmp/DecRate/Medusa5H1/MedusaHoligram/Medusa5H1 Part 2/Decimated-Rate FDP/Fdp/FreqDomainProcessing/CalculateAndApplyCoefficients/DeciRate/Calculate coefficients/StretchParamsTuning/Trivial Translation3 ==
  data: ESDUpperbounddBIn input; ESDUpperbounddB output; ESDLowerbounddB output; ESDLowerbounddBIn input; ESDStepSize output
  events: trigger input FUNCTION_CALL_EVENT
function [ESDUpperbounddB, ESDLowerbounddB, ESDStepSize]  = ...
                fcn(ESDUpperbounddBIn, ESDLowerbounddBIn)
            
if (ESDUpperbounddBIn.Value >= ESDLowerbounddBIn.Value)
    ESDUpperbounddB = ESDUpperbounddBIn.Value;
    ESDLowerbounddB = ESDLowerbounddBIn.Value;
else    
    TranslateError('Lower threshold for ESD cannot exceed upper threshold for ESD');
    ESDUpperbounddB = 0;
    ESDLowerbounddB = 0;
end

if (ESDUpperbounddBIn.Value == ESDLowerbounddBIn.Value)
    ESDStepSize = 0;
else
    ESDStepSize = 1/abs(ESDUpperbounddBIn.Value - ESDLowerbounddBIn.Value);
end

end

== matlab function Model_TranslationEngine64/ModelPreAmp/DecRate/Medusa5H1/MedusaHoligram/Medusa5H1 Part 2/Mono Detector/Mono Detector/Tune Translations/translation4 ==
  data: HPFNumStages output; HPFCutoff input; sampleRate input; HPFCoeffs output; numChannels parameter; maxNumStages parameter
  events: trigger input FUNCTION_CALL_EVENT
function [HPFNumStages, HPFCoeffs] = fcn(HPFCutoff, sampleRate, numChannels, maxNumStages)
%#codegen
%[Param:numChannels]
%[Param:maxNumStages]

% Calculation is fixed for a second order high pass butterworth, i.e. this 
% translation will not work anymore if the filter order/design is changed. 
% Code for computing hpf is taken from AR model.
% More generic implementation is also included below. In this case of 2nd 
% order filter, we get better precision by getting the one-stage sos 
% directly from the transfer function.

% hpfOrder = configStruct.hpfOrder;
% normFreq = 2 * HPFCutoff.Value / sampleRate;
% [Z, P, K] = butter_for_code_gen(hpfOrder, hpfOrder, normFreq, 'high');
% sos = zp2sos_for_code_gen(Z, P, K);

w = 2 * pi* HPFCutoff.Value / sampleRate;
sqrt2 = sqrt(2);
sinw = sin(w);
cosw = cos(w);

if (HPFCutoff.Value <= 0) || (HPFCutoff.Value > sampleRate/2)
    TranslateError('Highpass filter cutoff is out of range; should be in (0, %d)',sampleRate/2);
    b = single([1 0 0]);
    a = single([1 0 0]);
else
    denom = (sqrt2 + sinw);
    a1 = -2 * sqrt2 * cosw / denom;
    a2 = (sqrt2 - sinw) / denom;
    a = single([1 a1 a2]);
    b = single([1 -2 1] * (1-a1+a2) / 4);
end
sos = [b,a];

numStages = size(sos, 1) * ones(1, numChannels);
rawSOS = repmat(sos, numChannels, 1);

[HPFNumStages, HPFCoeffs] = pooliirTranslation(rawSOS, numStages, maxNumStages);

end


function [PoolNumStages, PoolCoeffs] = pooliirTranslation(rawSOS, numStages, maxNumStages)
% Function to format sos into pooliir. Taken from Translation block
% inside pooliir library block.

RawSOS = rawSOS;
NumStages = int32(numStages);
NumChannels = length(NumStages);

MaxNumStages = maxNumStages; 
PoolNumStages = int32(zeros(NumChannels,1));
PoolCoeffs = double(zeros(MaxNumStages * 4 + NumChannels,1));
ChannelCoeffs = zeros(MaxNumStages * 4 + 1,1);
ChannelSOS = double(zeros(MaxNumStages, 6));
SOSIndex = int32(0);

for i = 1:NumChannels
    
    ChannelNumStages = NumStages(i);   % Size of current SOS
    assert(ChannelNumStages <= MaxNumStages);
    
    ChannelSOS(1:ChannelNumStages,:) = RawSOS(SOSIndex+(1:ChannelNumStages),:);
    SOSIndex = SOSIndex + ChannelNumStages;

    if size(ChannelSOS,2) ~= 6
        TranslateError('SOS matrix must have 6 columns');
    end
    % decompose SOS
   
    ts = 1:4:4*ChannelNumStages;
    ChannelCoeffs(1,1) = prod(ChannelSOS(1:ChannelNumStages,1));        % b0
    
    % the remaining coeffs are compacted forms of the biquads
    ChannelCoeffs(1+ts,1) = ChannelSOS(1:ChannelNumStages,6);           % a2
    ChannelCoeffs(2+ts,1) = ChannelSOS(1:ChannelNumStages,5);           % a1
    if( ChannelSOS(:,1) == 0 )
    ChannelCoeffs(3+ts,1) = 0;                 % b2/b0
    ChannelCoeffs(4+ts,1) = 0;                 % b1/b0
    else
    ChannelCoeffs(3+ts,1) = ...
        ChannelSOS(1:ChannelNumStages,3)./ ...
        ChannelSOS(1:ChannelNumStages,1);  % b2/b0
    ChannelCoeffs(4+ts,1) = ...
        ChannelSOS(1:ChannelNumStages,2)./ ...
        ChannelSOS(1:ChannelNumStages,1);  % b1/b0
    end
    
    % length of Current Channel Coeffs
    ChannelCoeffsLength = 1+4*ChannelNumStages;
    
    % Offset into coefficient array for the current channel
    offset = (i-1)+4*sum(PoolNumStages(1:i-1));
    
    % Verify that the SOS does not violate the maximum number of stages
    % allocated for the pool
    PoolNumStages(i) = int32(ChannelNumStages);
    if sum(PoolNumStages) > MaxNumStages
        TranslateError('Too many second order sections');
    end

    % Store the coefficients
    PoolCoeffs(offset+(1:ChannelCoeffsLength)) = double(ChannelCoeffs(1:ChannelCoeffsLength));   
end
end

== matlab function Model_TranslationEngine64/ModelPreAmp/DecRate/Medusa5H1/MedusaHoligram/Medusa5H1 Part 3/On/Delay Tuning/Delay Translation/translation ==
  data: bassDelayDec output; wiggleDelay input; nearWiggleDelay input; bassDelayFull output; alignmentDelay output; DEC parameter; maxWiggleDelayDec parameter; maxNearWiggleDelayDec parameter; FDPDelay parameter; bandSplitDelay parameter; maxBassDelayFull parameter; maxBassDelayDec parameter; maxAlignmentDelay parameter
  events: trigger input FUNCTION_CALL_EVENT
function [bassDelayDec, bassDelayFull, alignmentDelay]  = fcn(wiggleDelay, nearWiggleDelay, DEC,...
                                                                maxWiggleDelayDec, maxNearWiggleDelayDec,...
                                                                FDPDelay, bandSplitDelay,...
                                                                maxBassDelayFull, maxBassDelayDec,...
                                                                maxAlignmentDelay)
%#codegen
%[Param:DEC]
%[Param:maxWiggleDelayDec]
%[Param:maxNearWiggleDelayDec]
%[Param:FDPDelay]
%[Param:bandSplitDelay]
%[Param:maxBassDelayFull]
%[Param:maxBassDelayDec]
%[Param:maxAlignmentDelay]

%% Alignment Delay Translation
% This translation computes the alignment delay values for bass and
% decimated-rate upmixed components

%% Error Check for incoming tune values
if(wiggleDelay.Value < 0)
    TranslateError('Value of ''Medusa Wiggle Delay'' must be greater than or equal to zero.');
end

if(nearWiggleDelay.Value < 0)
    TranslateError('Value of ''NEAR Wiggle Delay'' must be greater than or equal to zero.');
end

if(wiggleDelay.Value > maxWiggleDelayDec)
    TranslateError('Value of ''Medusa Wiggle Delay'' must be less than or equal to %d.', maxWiggleDelayDec);
end

if(nearWiggleDelay.Value > maxNearWiggleDelayDec)
    TranslateError('Value of ''NEAR Wiggle Delay'' must be less than or equal to %d.', maxNearWiggleDelayDec);
end

%% Computing the alignment delay values for bass and mid-range paths
% Medusa wiggle filter latency
wiggleDelayDec = int32(round(wiggleDelay.Value));
wiggleDelayFull = int32(wiggleDelayDec * DEC);

% NEAR wiggle filter latency
NEARWiggleDelayDec = int32(round(nearWiggleDelay.Value));
NEARWiggleDelayFull = int32(NEARWiggleDelayDec * DEC);

% Compute the bass alignment delay (applies to bass components)
actualBassDelay = FDPDelay + bandSplitDelay/2 + wiggleDelayFull + NEARWiggleDelayFull;
actualBassDelayDec = int32(floor(single(actualBassDelay)/DEC));
actualBassDelayFull = actualBassDelay - actualBassDelayDec*DEC;

% Compute the mid-range alignment delay (applies to decimated-rate upmixed components)
actualAlignmentDelay = wiggleDelayDec;

%% Error check for outgoing alignment delay values
if(actualBassDelayFull > maxBassDelayFull)
    TranslateError('Value of ''Medusa Bass Delay'' on decimated-rate path exceeds the maximum value of %d.', maxBassDelayFull);
end

if(actualBassDelayDec > maxBassDelayDec)
   TranslateError('Value of ''Medusa Bass Delay'' on full-rate path exceeds the maximum value of %d.', maxBassDelayDec);
end

if(actualAlignmentDelay > maxAlignmentDelay)
   TranslateError('Value of ''Medusa Alignment Delay'' on decimated-rate path exceeds the maximum value of %d.', maxAlignmentDelay);
end

%% Assigning outputs
bassDelayFull = actualBassDelayFull;
bassDelayDec = actualBassDelayDec;

alignmentDelay = actualAlignmentDelay;

end
